simulink model "desnutricion"  (Simulink 7.5)
settings: Solver=ode45  StartTime=0.0  StopTime=10.0  RelTol=1e-3
settings Model: Creator=My Laptop  LastModifiedBy=My Laptop

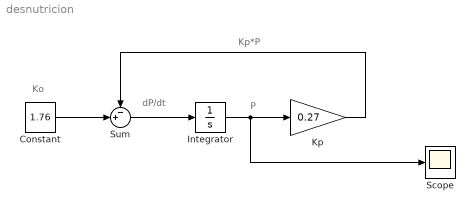
== system desnutricion ==
  note: P
  note: dP/dt
  note: Kp*P
  note: Ko
  Constant : Constant  Value=1.76  OutDataType=fixdt(1, 16)  OutScaling=2^0
  Integrator : Integrator  InitialCondition=234
  Kp : Gain  Gain=0.27  ParameterDataType=fixdt(1, 16)  ParameterScaling=2^0  OutDataType=fixdt(1, 16)  OutScaling=2^0
  Scope : Scope
  Sum : Sum  Inputs=-+|  OutDataType=fixdt(1, 16)  OutScaling=2^0
  wires:
  Integrator/1 -> Kp/1, Scope/1
  Kp/1 -> Sum/1
  Sum/1 -> Integrator/1
  Constant/1 -> Sum/2
